simulink model "BuildingModelWithSolarLoadAndHVAC"  (R2025a)
settings: Solver=daessc  StartTime=0.0  StopTime=604800  FixedStep=60*15  MaxStep=60  RelTol=1e-3  AbsTol=1e-3
PreLoadFcn:
  | % WallModelParams
libraries: nesl_utility x12, fl_lib x6, slpidlib x1
(part 1 of 2)
CloseFcn:
  | % clear flow out roomHeight wall win
settings Model: Creator=vikrants  LastModifiedBy=vikrants
settings SolverCC: AutoScaleAbsTol=off  NumberNewtonIterations=3.0  AlgebraicLoopSolver=TrustRegion  MaxZcPerStep=1.0
settings DebuggingCC: UnconnectedInputMsg=warning  UnconnectedOutputMsg=warning  UnconnectedLineMsg=warning  SymbolicDimsDataTypeCodeGenerationDiagnostic=none
settings ModelReferenceCC: EnableRefExpFcnMdlSchedulingChecks=on
settings SFSimCC: CustomCodeUndefinedFunction=UseInterfaceOnly
settings RTWCC: GPUComputeCapability=3.5  DLArmComputeVersion=19.05
settings SimscapeCC: SimscapeLogType=all  SimscapeLogSimulationStatistics=on  SimscapeLogDataHistory=10000.0  SimscapeMultithreadedCompilation=off

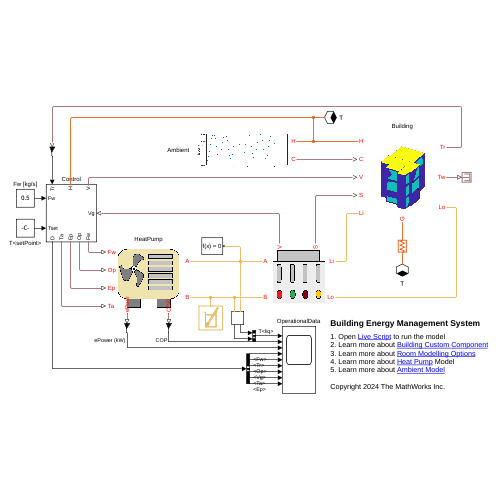
[thumbnail: Simulink's stored preview of the top-level diagram]
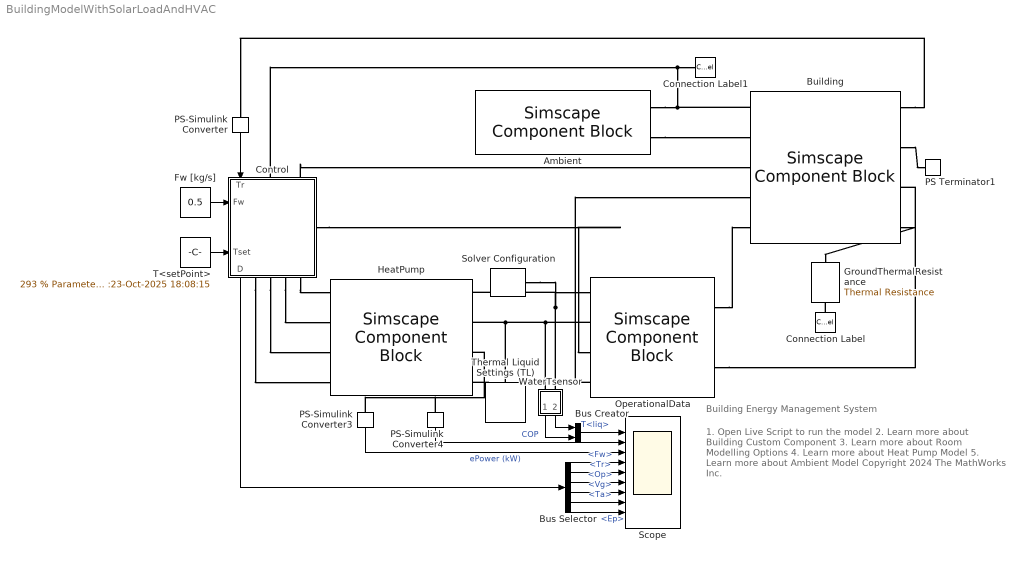
== system BuildingModelWithSolarLoadAndHVAC ==
  note: 1. Open Live Script to run the model
      | 2. Learn more about Building Custom Component
      | 3. Learn more about Room Modelling Options
      | 4. Learn more about Heat Pump Model
      | 5. Learn more about Ambient Model
      |
      | Copyright 2024 The MathWorks Inc.
  note: Building Energy Management System
  Ambient : SimscapeComponentBlock  SourceFile=EnvModel  ComponentPath=EnvModel  ComponentVariants="[\"EnvModel\"]"  ComponentVariantNames="[\"EnvModel\"]"  ClassName=EnvModel  SchemaVersion=1  listOfDays="[1  2  3  4  5  6  7] % Parameterized on :23-Oct-2025 18:08:15"  sunrise="[28933.8374      28933.0124      28929.4904      28923.2682      28914.3448      28902.7215       28888.402] % Parameterized on :23-Oct-2025 18:08:15 s"  sunset="[57466.1626      57466.9876      57470.5096      57476.7318      57485.6552      57497.2785       57511.598] % Parameterized on :23-Oct-2025 18:08:15 s"  startTime=3600 % Parameterized on :23-Oct-2025 18:08:15 s  avgDayTvec="[303  303  303  303  303  303  303] % Parameterized on :23-Oct-2025 18:08:15 K"  pcDayTvar=1 % Parameterized on :23-Oct-2025 18:08:15  avgNightTvec="[299  299  299  299  299  299  299] % Parameterized on :23-Oct-2025 18:08:15 K"  pcNightTvar=1 % Parameterized on :23-Oct-2025 18:08:15  cloudData=cloudCoverOptions.daily  cloudCoverVal="[0  0  0  0  0  0  0] % Parameterized on :23-Oct-2025 18:08:15"
      settings: CopyFcn=simscape.sscblock.internal.componentBlockCallback(gcbh,'COPY')  PreCopyFcn=simscape.sscblock.internal.componentBlockCallback(gcbh,'PRECOPY')  PreDeleteFcn=simscape.sscblock.internal.componentBlockCallback(gcbh,'PREDELETE')  InternalSimscapePortConfiguration="{\"Bottom\":[],\"Left\":[],\"Right\":[{\"id\":\"A\",\"label\":\"H\",\"type\":\"foundation.thermal.thermal\"},{\"id\":\"cloud\",\"label\":\"C\",\"type\":\"output\"}],\"Top\":[]}"
      mask Type: EnvModel
  Building : SimscapeComponentBlock  SourceFile=BuildingModel  ComponentPath=BuildingModel  ComponentVariants="[\"BuildingModel\"]"  ComponentVariantNames="[\"BuildingModel\"]"  ClassName=BuildingModel  SchemaVersion=1  nApts=3 % Parameterized on :23-Oct-2025 18:08:15  nRooms=5 % Parameterized on :23-Oct-2025 18:08:15  roomVolMat=[22.6534772736 39.6435852288 13.59208636416 9.9108963072 5.6633693184;22.6534772736 39.6435852288 13.59208636416 9.9108963072 5.6633693184;22.6534772736 39.6435852288 13.59208636416 9.9108963072 5.6633693184] % Parameterized on :23-Oct-2025 18:08:15 m^3  roomConnMat=[1 1 1 2 1.9235928 0.75;1 1 1 3 7.1789544 0.5;1 1 1 4 6.2816232 1;1 1 1 5 1.79493672 0.5;1 2 1 3 0.48121824 1;1 2 1 4 0.9614916 0.75;1 3 1 5 1.20210072 1;2 1 2 2 1.9235928 0.75;2 1 2 3 7.1789544 0.5;2 1 2 4 6.2816232 1;2 1 2 5 1.79493672 0.5;2 2 2 3 0.48121824 1;2 2 2 4 0.9614916 0.75;2 3 2 5 1.20210072 1;3 1 3 2 1.9235928 0.75;3 1 3 3 7.1789544 0.5;3 1 3 4 6.2816232 1;3 1 3 5 1.79493672 0.5;3 2 3 3 0.48121824 1;3 2 3 4 0.9614916 0.75;3 3 3 5 1.20210072 1] % Parameterized on :23-Oct-2025 18:08:15  floorConnMat=[1 1 2 1 7.43224 1;1 2 2 2 13.0064 1;1 3 2 3 4.45935 1;1 4 2 4 3.25161 1;1 5 2 5 1.85806 1;2 1 3 1 7.43224 1;2 2 3 2 13.0064 1;2 3 3 3 4.45935 1;2 4 3 4 3.25161 1;2 5 3 5 1.85806 1] % Parameterized on :23-Oct-2025 18:08:15  roomEnvConnMat=[1 1 1 2.22966 5.20254 0;1 1 2 1.393545 4.64515 0;1 1 4 1.85806 0 0;1 2 1 0 13.0064 0;1 2 2 9.2903 0 0;1 2 3 3.90192 9.10448 0;1 2 4 4.64515 4.64515 0;1 3 1 0.929051914 0 0;1 3 3 1.11484 3.90194 0;1 3 4 2.22966 5.20254 0;1 4 1 4.6452 0 0;1 4 2 4.55224 1.95096 0;1 4 3 0.92904 0 0;1 4 4 1.393570728 3.2516 0;1 5 1 4.6452 0 0;1 5 2 1.85805 0 0;1 5 3 0.92904 0 0;1 5 4 1.48644 2.22966 0;2 1 1 2.22966 5.20254 0;2 1 2 1.393545 4.64515 0;2 1 4 1.85806 0 0;2 2 1 0 13.0064 0;2 2 2 9.2903 0 0;2 2 3 3.90192 9.10448 0;2 2 4 4.64515 4.64515 0;2 3 1 0.929051914 0 0;2 3 3 1.11484 3.90194 0;2 3 4 2.22966 5.20254 0;2 4 1 4.6452 0 0;2 4 2 4.55224 1.95096 0;2 4 3 0.92904 0 0;2 4 4 1.393570728 3.2516 0;2 5 1 4.6452 0 0;2 5 2 1.85805 0 0;2 5 3 0.92904 0 0;2 5 4 1.48644 2.22966 0;3 1 1 2.22966 5.20254 0;3 1 2 1.393545 4.64515 0;3 1 4 1.85806 0 0;3 2 1 0 13.0064 0;3 2 2 9.2903 0 0;3 2 3 3.90192 9.10448 0;3 2 4 4.64515 4.64515 0;3 3 1 0.929051914 0 0;3 3 3 1.11484 3.90194 0;3 3 4 2.22966 5.20254 0;3 4 1 4.6452 0 0;3 4 2 4.55224 1.95096 0;3 4 3 0.92904 0 0;3 4 4 1.393570728 3.2516 0;3 5 1 4.6452 0 0;3 5 2 1.85805 0 0;3 5 3 0.92904 0 0;3 5 4 1.48644 2.22966 0] % Parameterized on :23-Oct-2025 18:08:15  roomEnvSolarRad=[0 0 0 0 0 0 0 0 0 0 0 93.65116 177.3749 198.6853 136.8637 0 0 0 0 0 0 0 0 0 0 0 0 0 0 0 0 0 0 0 0 94.86252 178.682 199.7233 137.414 0 0 0 0 0 0 0 0 0 0 0 0 0 0 0 0 0 0 0 0 96.10373 180.0564 200.8599 138.0853 0 0 0 0 0 0 0 0 0 0 0 0 0 0 0 0 0 0 0 0 97.37456 181.498 202.0955 138.8786 0 0 0 0 0 0 0 0 0 0 0 0 0 0 0 0 0 0 0 0 98.67471 183.0067 203.4304 139.7945 0 0 0 0 0 0 0 0 0 0 0 0 0 0 0 0 0 0 0 0 100.0039 184.5824 204.8647 140.834 0 0 0 0 0 0 0 0 0 0 0 0 0 0 0 0 0 0 0 0 101.3617 186.2247 206.3988 141.9976 0 0 0 0 0 0 0 0 0 0;0 0 0 0 0 0 0 0 0 0 0 0 0 0 0 0 0 0 0 0 0 0 0 0 0 0 0 0 0 0 0 0 0 0 0 0 0 0 0 0 0 0 0 0 0 0 0 0 0 0 0 0 0 0 0 0 0 0 0 0 0 0 0 0 0 0 0 0 0 0 0 0 0 0 0 0 0 0 0 0 0 0 0 0 0 0 0 0 0 0 0 0 0 0 0 0 0 0 0 0 0 0 0 0 0 0 0 0 0 0 0 0 0 0 0 0 0 0 0 0 0 0 0 0 0 0 0 0 0 0 0 0 0 0 0 0 0 0 0 0 0 0 0 0 0 0 0 0 0 0 0 0 0 0 0 0 0 0 0 0 0 0 0 0 0 0 0 0 0;0 0 0 0 0 0 0 0 142.8462 239.0062 293.6475 287.8589 224.8602 132.4751 48.80781 0 0 0 0 0 0 0 0 0 0 0 0 0 0 0 0 0 144.7366 240.8153 295.1148 288.755 225.1512 132.3647 48.62846 0 0 0 0 0 0 0 0 0 0 0 0 0 0 0 0 0 146.7023 242.7125 296.6788 289.7448 225.5201 132.3084 48.48171 0 0 0 0 0 0 0 0 0 0 0 0 0 0 0 0 0 148.7418 244.6967 298.3387 290.8281 225.9666 132.3058 48.36703 0 0 0 0 0 0 0 0 0 0 0 0 0 0 0 0 0 150.8536 246.7667 300.0937 292.0043 226.4904 132.3564 48.28381 0 0 0 0 0 0 0 0 0 0 0 0 0 0 0 0 0 153.0361 248.9213 301.9431 293.273 227.0912 132.4599 48.23142 0 0 0 0 0 0 0 0 0 0 0 0 0 0 0 0 0 155.2877 251.1593 303.886 294.6337 227.7686 132.6158 48.20913 0 0 0 0 0 0 0 0 0 0;0 0 0 0 0 0 0 0 0 0 0 93.65116 177.3749 198.6853 136.8637 0 0 0 0 0 0 0 0 0 0 0 0 0 0 0 0 0 0 0 0 94.86252 178.682 199.7233 137.414 0 0 0 0 0 0 0 0 0 0 0 0 0 0 0 0 0 0 0 0 96.10373 180.0564 200.8599 138.0853 0 0 0 0 0 0 0 0 0 0 0 0 0 0 0 0 0 0 0 0 97.37456 181.498 202.0955 138.8786 0 0 0 0 0 0 0 0 0 0 0 0 0 0 0 0 0 0 0 0 98.67471 183.0067 203.4304 139.7945 0 0 0 0 0 0 0 0 0 0 0 0 0 0 0 0 0 0 0 0 100.0039 184.5824 204.8647 140.834 0 0 0 0 0 0 0 0 0 0 0 0 0 0 0 0 0 0 0 0 101.3617 186.2247 206.3988 141.9976 0 0 0 0 0 0 0 0 0 0;0 0 0 0 0 0 0 0 0 0 0 0 0 0 0 0 0 0 0 0 0 0 0 0 0 0 0 0 0 0 0 0 0 0 0 0 0 0 0 0 0 0 0 0 0 0 0 0 0 0 0 0 0 0 0 0 0 0 0 0 0 0 0 0 0 0 0 0 0 0 0 0 0 0 0 0 0 0 0 0 0 0 0 0 0 0 0 0 0 0 0 0 0 0 0 0 0 0 0 0 0 0 0 0 0 0 0 0 0 0 0 0 0 0 0 0 0 0 0 0 0 0 0 0 0 0 0 0 0 0 0 0 0 0 0 0 0 0 0 0 0 0 0 0 0 0 0 0 0 0 0 0 0 0 0 0 0 0 0 0 0 0 0 0 0 0 0 0 0;0 0 0 0 0 0 0 0 0 0 0 0 0 0 0 0 0 0 0 0 0 0 0 0 0 0 0 0 0 0 0 0 0 0 0 0 0 0 0 0 0 0 0 0 0 0 0 0 0 0 0 0 0 0 0 0 0 0 0 0 0 0 0 0 0 0 0 0 0 0 0 0 0 0 0 0 0 0 0 0 0 0 0 0 0 0 0 0 0 0 0 0 0 0 0 0 0 0 0 0 0 0 0 0 0 0 0 0 0 0 0 0 0 0 0 0 0 0 0 0 0 0 0 0 0 0 0 0 0 0 0 0 0 0 0 0 0 0 0 0 0 0 0 0 0 0 0 0 0 0 0 0 0 0 0 0 0 0 0 0 0 0 0 0 0 0 0 0 0;0 0 0 0 0 0 0 0 142.8462 239.0062 293.6475 287.8589 224.8602 132.4751 48.80781 0 0 0 0 0 0 0 0 0 0 0 0 0 0 0 0 0 144.7366 240.8153 295.1148 288.755 225.1512 132.3647 48.62846 0 0 0 0 0 0 0 0 0 0 0 0 0 0 0 0 0 146.7023 242.7125 296.6788 289.7448 225.5201 132.3084 48.48171 0 0 0 0 0 0 0 0 0 0 0 0 0 0 0 0 0 148.7418 244.6967 298.3387 290.8281 225.9666 132.3058 48.36703 0 0 0 0 0 0 0 0 0 0 0 0 0 0 0 0 0 150.8536 246.7667 300.0937 292.0043 226.4904 132.3564 48.28381 0 0 0 0 0 0 0 0 0 0 0 0 0 0 0 0 0 153.0361 248.9213 301.9431 293.273 227.0912 132.4599 48.23142 0 0 0 0 0 0 0 0 0 0 0 0 0 0 0 0 0 155.2877 251.1593 303.886 294.6337 227.7686 132.6158 48.20913 0 0 0 0 0 0 0 0 0 0;0 0 0 0 0 0 0 0 0 0 0 93.65116 177.3749 198.6853 136.8637 0 0 0 0 0 0 0 0 0 0 0 0 0 0 0 0 0 0 0 0 94.86252 178.682 199.7233 137.414 0 0 0 0 0 0 0 0 0 0 0 0 0 0 0 0 0 0 0 0 96.10373 180.0564 200.8599 138.0853 0 0 0 0 0 0 0 0 0 0 0 0 0 0 0 0 0 0 0 0 97.37456 181.498 202.0955 138.8786 0 0 0 0 0 0 0 0 0 0 0 0 0 0 0 0 0 0 0 0 98.67471 183.0067 203.4304 139.7945 0 0 0 0 0 0 0 0 0 0 0 0 0 0 0 0 0 0 0 0 100.0039 184.5824 204.8647 140.834 0 0 0 0 0 0 0 0 0 0 0 0 0 0 0 0 0 0 0 0 101.3617 186.2247 206.3988 141.9976 0 0 0 0 0 0 0 0 0 0;0 0 0 0 0 0 0 0 0 0 0 0 0 0 0 0 0 0 0 ...(+22234 chars)] % Parameterized on :23-Oct-2025 18:08:15  floorGroundConn=[1 1 7.4322432;1 2 13.0064256;1 3 4.45934592;1 4 3.2516064;1 5 1.8580608] % Parameterized on :23-Oct-2025 18:08:15  roomModelOption=roomPhysicsOptions.roomRadiatorUF  roomRadiatorArea=[2.322576 3.2516064 1.8580608 1.6258032 1.161288;2.322576 3.2516064 1.8580608 1.6258032 1.161288;2.322576 3.2516064 1.8580608 1.6258032 1.161288] % Parameterized on :23-Oct-2025 18:08:15 m^2  roomUFPipingArea=[7.4322432 13.0064256 4.013411328 2.92644576 1.8580608;7.4322432 13.0064256 4.013411328 2.92644576 1.8580608;7.4322432 13.0064256 4.013411328 2.92644576 1.8580608] % Parameterized on :23-Oct-2025 18:08:15 m^2  roofEnvConnMat=[3 1 7.4322432;3 2 13.0064256;3 3 4.45934592;3 4 3.2516064;3 5 1.8580608] % Parameterized on :23-Oct-2025 18:08:15  roofEnvSolarRad=[0 0 0 0 0 0 0 0 135.3688 244.6002 318.0249 338.3299 301.6173 215.2339 101.2105 0 0 0 0 0 0 0 0 0 0 0 0 0 0 0 0 0 137.349 246.6202 319.7841 339.6663 302.4684 215.6179 101.2704 0 0 0 0 0 0 0 0 0 0 0 0 0 0 0 0 0 139.4098 248.7357 321.6488 341.1138 303.4312 216.1063 101.4179 0 0 0 0 0 0 0 0 0 0 0 0 0 0 0 0 0 141.55 250.9457 323.6182 342.672 304.5056 216.6994 101.653 0 0 0 0 0 0 0 0 0 0 0 0 0 0 0 0 0 143.7687 253.249 325.6913 344.3403 305.6916 217.3972 101.9758 0 0 0 0 0 0 0 0 0 0 0 0 0 0 0 0 0 146.0648 255.6446 327.8673 346.1181 306.9889 218.1999 102.3866 0 0 0 0 0 0 0 0 0 0 0 0 0 0 0 0 0 148.4371 258.1313 330.1451 348.0048 308.3973 219.1077 102.8853 0 0 0 0 0 0 0 0 0 0;0 0 0 0 0 0 0 0 135.3688 244.6002 318.0249 338.3299 301.6173 215.2339 101.2105 0 0 0 0 0 0 0 0 0 0 0 0 0 0 0 0 0 137.349 246.6202 319.7841 339.6663 302.4684 215.6179 101.2704 0 0 0 0 0 0 0 0 0 0 0 0 0 0 0 0 0 139.4098 248.7357 321.6488 341.1138 303.4312 216.1063 101.4179 0 0 0 0 0 0 0 0 0 0 0 0 0 0 0 0 0 141.55 250.9457 323.6182 342.672 304.5056 216.6994 101.653 0 0 0 0 0 0 0 0 0 0 0 0 0 0 0 0 0 143.7687 253.249 325.6913 344.3403 305.6916 217.3972 101.9758 0 0 0 0 0 0 0 0 0 0 0 0 0 0 0 0 0 146.0648 255.6446 327.8673 346.1181 306.9889 218.1999 102.3866 0 0 0 0 0 0 0 0 0 0 0 0 0 0 0 0 0 148.4371 258.1313 330.1451 348.0048 308.3973 219.1077 102.8853 0 0 0 0 0 0 0 0 0 0;0 0 0 0 0 0 0 0 135.3688 244.6002 318.0249 338.3299 301.6173 215.2339 101.2105 0 0 0 0 0 0 0 0 0 0 0 0 0 0 0 0 0 137.349 246.6202 319.7841 339.6663 302.4684 215.6179 101.2704 0 0 0 0 0 0 0 0 0 0 0 0 0 0 0 0 0 139.4098 248.7357 321.6488 341.1138 303.4312 216.1063 101.4179 0 0 0 0 0 0 0 0 0 0 0 0 0 0 0 0 0 141.55 250.9457 323.6182 342.672 304.5056 216.6994 101.653 0 0 0 0 0 0 0 0 0 0 0 0 0 0 0 0 0 143.7687 253.249 325.6913 344.3403 305.6916 217.3972 101.9758 0 0 0 0 0 0 0 0 0 0 0 0 0 0 0 0 0 146.0648 255.6446 327.8673 346.1181 306.9889 218.1999 102.3866 0 0 0 0 0 0 0 0 0 0 0 0 0 0 0 0 0 148.4371 258.1313 330.1451 348.0048 308.3973 219.1077 102.8853 0 0 0 0 0 0 0 0 0 0;0 0 0 0 0 0 0 0 135.3688 244.6002 318.0249 338.3299 301.6173 215.2339 101.2105 0 0 0 0 0 0 0 0 0 0 0 0 0 0 0 0 0 137.349 246.6202 319.7841 339.6663 302.4684 215.6179 101.2704 0 0 0 0 0 0 0 0 0 0 0 0 0 0 0 0 0 139.4098 248.7357 321.6488 341.1138 303.4312 216.1063 101.4179 0 0 0 0 0 0 0 0 0 0 0 0 0 0 0 0 0 141.55 250.9457 323.6182 342.672 304.5056 216.6994 101.653 0 0 0 0 0 0 0 0 0 0 0 0 0 0 0 0 0 143.7687 253.249 325.6913 344.3403 305.6916 217.3972 101.9758 0 0 0 0 0 0 0 0 0 0 0 0 0 0 0 0 0 146.0648 255.6446 327.8673 346.1181 306.9889 218.1999 102.3866 0 0 0 0 0 0 0 0 0 0 0 0 0 0 0 0 0 148.4371 258.1313 330.1451 348.0048 308.3973 219.1077 102.8853 0 0 0 0 0 0 0 0 0 0;0 0 0 0 0 0 0 0 135.3688 244.6002 318.0249 338.3299 301.6173 215.2339 101.2105 0 0 0 0 0 0 0 0 0 0 0 0 0 0 0 0 0 137.349 246.6202 319.7841 339.6663 302.4684 215.6179 101.2704 0 0 0 0 0 0 0 0 0 0 0 0 0 0 0 0 0 139.4098 248.7357 321.6488 341.1138 303.4312 216.1063 101.4179 0 0 0 0 0 0 0 0 0 0 0 0 0 0 0 0 0 141.55 250.9457 323.6182 342.672 304.5056 216.6994 101.653 0 0 0 0 0 0 0 0 0 0 0 0 0 0 0 0 0 143.7687 253.249 325.6913 344.3403 305.6916 217.3972 101.9758 0 0 0 0 0 0 0 0 0 0 0 0 0 0 0 0 0 146.0648 255.6446 327.8673 346.1181 306.9889 218.1999 102.3866 0 0 0 0 0 0 0 0 0 0 0 0 0 0 0 0 0 148.4371 258.1313 330.1451 348.0048 308.3973 219.1077 102.8853 0 0 0 0 0 0 0 0 0 0] % Parameterized on :23-Oct-2025 18:08:15  radiatorPipeGap=1e-2 m  radiatorPipeHydrDia=0.022 m  radiatorPipeArea=pi*(0.022^2)/4 m^2  UFPipeGap=1e-2 m  UFPipeHydrDia=0.015 m  UFPipeArea=pi*(0.015^2)/4 m^2  wallPropValue=wallPhysicsOptions.allWallNotSame  wallAbsorptivityValue=0.6  wallThicknessValue=.3 m  wallMaterialDenValue=2400 kg/m^3  wallMaterialCpValue=750 J/(K*kg)  wallThermalKValue=2 W/(K*m)  extWallAbsorptivityVal=0.6 % Parameterized on :23-Oct-2025 18:08:15  extWallThicknessVal=0.3 % Parameterized on :23-Oct-2025 18:08:15 m  extWallMaterialDenVal=2400 % Parameterized on :23-Oct-2025 18:08:15 kg/m^3  extWallMaterialCpVal=750 % Parameterized on :23-Oct-2025 18:08:15 J/(K*kg)  extWallThermalKVal=2 % Parameterized on :23-Oct-2025 18:08:15 W/(K*m)  intWallThicknessVal=0.3 % Parameterized on :23-Oct-2025 18:08:15 m  intWallMaterialDenVal=2400 % Parameterized on :23-Oct-2025 18:08:15 kg/m^3  intWallMaterialCpVal=750 % Parameterized on :23-Oct-2025 18:08:15 J/(K*kg)  intWallThermalKVal=2 % Parameterized on :23-Oct-2025 18:08:15 W/(K*m)  intFloorThicknessVal=0.3 % Parameterized on :23-Oct-2025 18:08:15 m  intFloorMaterialDenVal=2400 % Parameterized on :23-Oct-2025 18:08:15 kg/m^3  intFloorMaterialCpVal=750 % Parameterized on :23-Oct-2025 18:08:15 J/(K*kg)  intFloorThermalKVal=2 % Parameterized on :23-Oct-2025 18:08:15 W/(K*m)  roofAbsorptivityVal=0.6 % Parameterized on :23-Oct-2025 18:08:15  roofThicknessVal=0.3 % Parameterized on :23-Oct-2025 18:08:15 m  roofMaterialDenVal=2400 % Parameterized on :23-Oct-2025 18:08:15 kg/m^3  roofMaterialCpVal=750 % Parameterized on :23-Oct-2025 18:08:15 J/(K*kg)  roofThermalKVal=2 % Parameterized on :23-Oct-2025 18:08:15 W/(K*m)  winAbsorptivity=0.4 % Parameterized on :23-Oct-2025 18:08:15  winTransmissivity=0.2 % Parameterized on :23-Oct-2025 18:08:15  winThickness=0.01 % Parameterized on :23-Oct-2025 18:08:15 m  winMaterialDen=4000 % Parameterized on :23-Oct-2025 18:08:15 kg/m^3  winMaterialCp=840 % Parameterized on :23-Oct-2025 18:08:15 J/(K*kg)  winThermalK=1 % Parameterized on :23-Oct-2025 18:08:15 W/(K*m)  heatTransferPipeRoughness=1e-06 m  extToWallHTC=50 % Parameterized on :23-Oct-2025 18:08:15 W/(K*m^2)  intToRoomHTC=25 % Parameterized on :23-Oct-2025 18:08:15 W/(K*m^2)  iniTemperature=294.1 % Parameterized on :23-Oct-2025 18:08:15 K  airDensity=1.28 kg/m^3  airCp=700 J/(K*kg)  minArea=1e-10 m^2
      settings: CopyFcn=simscape.sscblock.internal.componentBlockCallback(gcbh,'COPY')  PreCopyFcn=simscape.sscblock.internal.componentBlockCallback(gcbh,'PRECOPY')  PreDeleteFcn=simscape.sscblock.internal.componentBlockCallback(gcbh,'PREDELETE')  InternalSimscapePortConfiguration="{\"Bottom\":[{\"id\":\"G\",\"label\":\"G\",\"type\":\"foundation.thermal.thermal\"}],\"Left\":[{\"id\":\"H\",\"label\":\"H\",\"type\":\"foundation.thermal.thermal\"},{\"id\":\"C\",\"label\":\"C\",\"type\":\"input\"},{\"id\":\"V\",\"label\":\"V\",\"type\":\"input\"},{\"id\":\"S\",\"label\":\"S\",\"type\":\"input\"},{\"id\":\"A\",\"label\":\"Li\",\"type\":\"foundation.thermal_liquid.thermal_liquid\"}],\"Right\":[{\"id\":\"roomTemp\",\"label\":\"Tr\",\"type\":\"output\"},{\"id\":\"wallTemp\",\"label\":\"Tw\",\"type\":\"output\"},{\"id\":\"B\",\"label\":\"Lo\",\"type\":\"foundation.thermal_liquid.thermal_liquid\"}],\"Top\":[]}"
      mask Type: BuildingModel
  Bus Creator : BusCreator  Inputs=2
  Bus Selector : BusSelector  OutputSignals=Fw,Tr,Op,Vg,Ta,Ep
  Connection Label : ConnectionLabel  Label=T
  Connection Label1 : ConnectionLabel  Label=T
  Control : Subsystem
      settings: PortSchema="{\"entries\":[{\"content\":{\"sides\":[{\"content\":{\"connectorIds\":[\"LConn1\"]},\"type\":\"ConnectorPlacement.EquallySpacedRectSide\",\"uuid\":\"3ed745ff-0b79-4fb7-8a1a-34583b4b790f\"},{\"content\":{\"connectorIds\":[\"In2\",\"In3\"],\"side\":\"RIGHT\"},\"type\":\"ConnectorPlacement.EquallySpacedRectSide\",\"uuid\":\"620bee4e-94f2-4040-b1cd-05a3221b3be9\"},{\"content\":{\"connectorIds\":[\"LConn2\",\"LConn3\",\"LConn4\",\"LConn5\",\"Out1\"],\"side\":\"TOP\"},\"type\":\"ConnectorPlacement.EquallySpacedRectSide\",\"uuid\":\"f68ff0b5-8e3a-4982-a173-63d19766a609\"},{\"content\":{\"connectorIds\":[\"RConn1\",\"RConn2\",\"In1\"],\"side\":\"BOTTOM\"},\"type\":\"ConnectorPlacement.EquallySpacedRectSide\",\"uuid\":\"2c8538cc-0234-4c65-909e-07f5b83fead8\"}]},\"type\":\"ConnectorPlacement.EquallySpacedConnector\",\"uuid\":\"126dfa7a-8255-403e-a375-633719ca790e\"}],\"packageUris\":[\"http://schema.mathworks.com/mf0/Connector/R2020b\"],\"version\":\"1.0\"}"
  Fw [kg/s] : Constant  Value=0.5
  GroundThermalResistance : fl_lib/Thermal/Thermal Elements/Thermal Resistance  resistance=100 % Parameterized on :23-Oct-2025 18:08:15 K/W  T_specify=off  T_priority=None  T=0 K  T_nominal_specify=off  T_nominal_value=1  T_nominal_unit=K  Q_specify=off  Q_priority=None  Q=0 W  Q_nominal_specify=off  Q_nominal_value=1  Q_nominal_unit=W
  HeatPump : SimscapeComponentBlock  SourceFile=HeatPumpModel  ComponentPath=HeatPumpModel  ComponentVariants="[\"HeatPumpModel\"]"  ComponentVariantNames="[\"HeatPumpModel\"]"  ClassName=HeatPumpModel  SchemaVersion=1  heatingCapacityA=10.17 kW  heatingCoPA=4.86  heatingCapacityB=10.12 kW  heatingCoPB=3.7  heatingCapacityC=10.17 kW  heatingCoPC=4.86  heatingCapacityD=10.12 kW  heatingCoPD=3.7  coolingCapacityE=10.55 kW  coolingCoPE=4.13  coolingCapacityF=6.9 kW  coolingCoPF=2.7  elecHeaterPower=2 kW  coilLen=1 m  coilDia=.05 m  coilArea=pi*(0.05^2)/4 m^2  initialT=299.8 K  initialP=.101325*2 MPa  expansionVol=0.01 m^3  nomDevOption=NominalConditionDeviationModel.enabled  modelOption=HeatPumpOptions.singleUnit  numHeatPumps=3  nominalFlow=0.5 kg/s  minWaterFlowRate=1e-3 kg/s  measTimelag=6 s  waterOpTempMin=281 K  waterOpTempMax=345 K  waterSpHeat=[4183, 4187, 4180, 4180, 4180, 4195] J/(K*kg)
      settings: CopyFcn=simscape.sscblock.internal.componentBlockCallback(gcbh,'COPY')  PreCopyFcn=simscape.sscblock.internal.componentBlockCallback(gcbh,'PRECOPY')  PreDeleteFcn=simscape.sscblock.internal.componentBlockCallback(gcbh,'PREDELETE')  InternalSimscapePortConfiguration="{\"Bottom\":[{\"id\":\"ePow\",\"label\":\"ePow\",\"type\":\"output\"},{\"id\":\"COP\",\"label\":\"COP\",\"type\":\"output\"}],\"Left\":[{\"id\":\"Fw\",\"label\":\"Fw\",\"type\":\"input\"},{\"id\":\"Op\",\"label\":\"Op\",\"type\":\"input\"},{\"id\":\"Ep\",\"label\":\"Ep\",\"type\":\"input\"},{\"id\":\"Ta\",\"label\":\"Ta\",\"type\":\"input\"}],\"Right\":[{\"id\":\"A\",\"label\":\"A\",\"type\":\"foundation.thermal_liquid.thermal_liquid\"},{\"id\":\"B\",\"label\":\"B\",\"type\":\"foundation.thermal_liquid.thermal_liquid\"}],\"Top\":[]}"
      mask Type: HeatPumpModel
  OperationalData : SimscapeComponentBlock  SourceFile=BuildingHVACOperation  ComponentPath=BuildingHVACOperation  ComponentVariants="[\"BuildingHVACOperation\"]"  ComponentVariantNames="[\"BuildingHVACOperation\"]"  ClassName=BuildingHVACOperation  SchemaVersion=1  roomModelOption=roomPhysicsOptions.roomRadiatorUF  opsParamBldg=[1 1 1 1 0 0 0;1 1 2 1 0 0 0;1 1 3 1 0 0 0;1 1 4 1 0 0 0;1 1 5 1 0 0 0;2 2 1 1 0 0 0;2 2 2 1 0 0 2;2 2 3 1 0 0 0;2 2 4 1 0 0 0;2 2 5 1 0 0 0;3 3 1 1 0 0 0;3 3 2 1 0 0 0;3 3 3 1 0 0 0;3 3 4 1 0 0 0;3 3 5 1 0 0 0;1 1 1 1 0 0 0;1 1 2 1 0 0 0;1 1 3 1 0 0 0;1 1 4 1 0 0 0;1 1 5 1 0 0 0;2 2 1 1 0 0 0;2 2 2 1 0 0 2;2 2 3 1 0 0 0;2 2 4 1 0 0 0;2 2 5 1 0 0 0;3 3 1 1 0 0 0;3 3 2 1 0 0 0;3 3 3 1 0 0 0;3 3 4 1 0 0 0;3 3 5 1 0 0 0;1 1 1 1 0 0 0;1 1 2 1 0 0 0;1 1 3 1 0 0 0;1 1 4 1 0 0 0;1 1 5 1 0 0 0;2 2 1 1 0 0 0;2 2 2 1 0 0 2;2 2 3 1 0 0 0;2 2 4 1 0 0 0;2 2 5 1 0 0 0;3 3 1 1 0 0 0;3 3 2 1 0 0 0;3 3 3 1 0 0 0;3 3 4 1 0 0 0;3 3 5 1 0 0 0;1 1 1 1 0 0 1;1 1 2 1 0 0 0;1 1 3 1 0 0 0;1 1 4 1 0 0 0;1 1 5 1 0 0 0;2 2 1 1 0 0 0;2 2 2 1 0 0 0;2 2 3 1 0 0 0;2 2 4 1 0 0 0;2 2 5 1 0 0 0;3 3 1 1 0 0 0;3 3 2 1 0 0 0;3 3 3 1 0 0 0;3 3 4 1 0 0 0;3 3 5 1 0 0 0;1 1 1 1 0 0 1;1 1 2 1 0 0 0;1 1 3 1 0 0 0;1 1 4 1 0 0 0;1 1 5 1 0 0 0;2 2 1 1 0 0 0;2 2 2 1 0 0 0;2 2 3 1 0 0 0;2 2 4 1 0 0 0;2 2 5 1 0 0 0;3 3 1 1 0 0 0;3 3 2 1 0 0 0;3 3 3 1 0 0 0;3 3 4 1 0 0 0;3 3 5 1 0 0 0;1 1 1 1 0 0 1;1 1 2 1 0 0 0;1 1 3 1 0 0 0;1 1 4 1 0 0 0;1 1 5 1 0 0 0;2 2 1 1 0 0 0;2 2 2 1 0 0 0;2 2 3 1 0 0 0;2 2 4 1 0 0 0;2 2 5 1 0 0 0;3 3 1 1 0 0 0;3 3 2 1 0 0 0;3 3 3 1 0 0 0;3 3 4 1 0 0 0;3 3 5 1 0 0 0;1 1 1 0 0 0 0;1 1 2 0 0 0 0;1 1 3 0 0 0 0;1 1 4 0 0 0 0;1 1 5 1 0 0 0;2 2 1 0 0 0 0;2 2 2 0 0 0 0;2 2 3 0 0 0 0;2 2 4 0 0 0 0;2 2 5 1 0 0 0;3 3 1 0 0 0 0;3 3 2 0 0 0 0;3 3 3 0 0 0 0;3 3 4 0 0 0 0;3 3 5 1 0 0 0;1 1 1 0 0 0 0;1 1 2 0 0 0 0;1 1 3 0 0 0 0;1 1 4 0 0 0 0;1 1 5 1 0 0 0;2 2 1 0 0 0 0;2 2 2 0 0 0 0;2 2 3 0 0 0 0;2 2 4 0 0 0 0;2 2 5 1 0 0 0;3 3 1 0 0 0 0;3 3 2 0 0 0 0;3 3 3 0 0 0 0;3 3 4 0 0 0 0;3 3 5 1 0 0 0;1 1 1 0 0 0 0;1 1 2 0 0 0 0;1 1 3 0 0 0 0;1 1 4 0 0 0 0;1 1 5 1 0 0 0;2 2 1 0 0 0 0;2 2 2 0 0 0 0;2 2 3 0 0 0 0;2 2 4 0 0 0 0;2 2 5 1 0 0 0;3 3 1 0 0 0 0;3 3 2 0 0 0 0;3 3 3 0 0 0 0;3 3 4 0 0 0 0;3 3 5 1 0 0 0;1 1 1 0 0 0 0;1 1 2 0 0 0 0;1 1 3 0 0 0 0;1 1 4 0 0 0 0;1 1 5 1 0 0 0;2 2 1 0 0 0 0;2 2 2 0 0 0 0;2 2 3 0 0 0 0;2 2 4 0 0 0 0;2 2 5 1 0 0 0;3 3 1 0 0 0 0;3 3 2 0 0 0 0;3 3 3 0 0 0 0;3 3 4 0 0 0 0;3 3 5 1 0 0 0;1 1 1 0 0 0 0;1 1 2 0 0 0 0;1 1 3 0 0 0 0;1 1 4 0 0 0 0;1 1 5 1 0 0 0;2 2 1 0 0 0 0;2 2 2 0 0 0 0;2 2 3 0 0 0 0;2 2 4 0 0 0 0;2 2 5 1 0 0 0;3 3 1 0 0 0 0;3 3 2 0 0 0 0;3 3 3 0 0 0 0;3 3 4 0 0 0 0;3 3 5 1 0 0 0;1 1 1 0 0 0 0;1 1 2 0 0 0 0;1 1 3 0 0 0 0;1 1 4 0 0 0 0;1 1 5 1 0 0 0;2 2 1 0 0 0 0;2 2 2 0 0 0 0;2 2 3 0 0 0 0;2 2 4 0 0 0 0;2 2 5 1 0 0 0;3 3 1 0 0 0 0;3 3 2 0 0 0 0;3 3 3 0 0 0 0;3 3 4 0 0 0 0;3 3 5 1 0 0 0;1 1 1 0 0 0 0;1 1 2 0 0 0 0;1 1 3 0 0 0 0;1 1 4 0 0 0 0;1 1 5 1 0 0 0;2 2 1 0 0 0 0;2 2 2 0 0 0 0;2 2 3 0 0 0 0;2 2 4 0 0 0 0;2 2 5 1 0 0 0;3 3 1 0 0 0 0;3 3 2 0 0 0 0;3 3 3 0 0 0 0;3 3 4 0 0 0 0;3 3 5 1 0 0 0;1 1 1 1 0 0 0;1 1 2 1 0 0 0;1 1 3 1 0 0 0;1 1 4 1 0 0 0;1 1 5 1 0 0 0;2 2 1 1 0 0 0;2 2 2 1 0 0 0;2 2 3 1 0 0 0;2 2 4 1 0 0 0;2 2 5 1 0 0 0;3 3 1 1 0 0 0;3 3 2 1 0 0 0;3 3 3 1 0 0 2;3 3 4 1 0 0 0;3 3 5 1 0 0 0;1 1 1 1 0 0 0;1 1 2 1 0 0 0;1 1 3 1 0 0 0;1 1 4 1 0 0 0;1 1 5 1 0 0 0;2 2 1 1 0 0 0;2 2 2 1 0 0 2;2 2 3 1 0 0 0;2 2 4 1 0 0 0;2 2 5 1 0 0 0;3 3 1 1 0 0 0;3 3 2 1 0 0 0;3 3 3 1 0 0 0;3 3 4 1 0 0 0;3 3 5 1 0 0 0;1 1 1 1 0 0 0;1 1 2 1 0 0 0;1 1 3 1 0 0 0;1 1 4 1 0 0 0;1 1 5 1 0 0 0;2 2 1 1 0 0 0;2 2 2 1 0 0 2;2 2 3 1 0 0 0;2 2 4 1 0 0 0;2 2 5 1 0 0 0;3 3 1 1 0 0 0;3 3 2 1 0 0 0;3 3 3 1 0 0 0;3 3 4 1 0 0 0;3 3 5 1 0 0 0;1 1 1 1 0 0 0;1 1 2 1 0 0 0;1 1 3 1 0 0 0;1 1 4 1 0 0 0;1 1 5 1 0 0 0;2 2 1 1 0 0 0;2 2 2 1 0 0 2;2 2 3 1 0 0 0;2 2 4 1 0 0 0;2 2 5 1 0 0 0;3 3 1 1 0 0 0;3 3 2 1 0 0 0;3 3 3 1 0 0 0;3 3 4 1 0 0 0;3 3 5 1 0 0 0;1 1 1 1 0 0 0;1 1 2 1 0 0 0;1 1 3 1 0 0 0;1 1 4 1 0 0 0;1 1 5 1 0 0 0;2 2 1 1 0 0 0;2 2 2 1 0 0 2;2 2 3 1 0 0 0;2 2 4 1 0 0 0;2 2 5 1 0 0 0;3 3 1 1 0 0 0;3 3 2 1 0 0 0;3 3 3 1 0 0 0;3 3 4 1 0 0 0;3 3 5 1 0 0 0;1 1 1 1 0 0 0;1 1 2 1 0 0 0;1 1 3 1 0 0 0;1 1 4 1 0 0 0;1 1 5 1 0 0 0;2 2 1 1 0 0 0;2 2 2 1 0 0 2;2 2 3 1 0 0 0;2 2 4 1 0 0 0;2 2 5 1 0 0 0;3 3 1 1 0 0 0;3 3 2 1 0 0 0;3 3 3 1 0 0 0;3 3 4 1 0 0 0;3 3 5 1 0 0 0;1 1 1 1 ...(+31492 chars)] % Parameterized on :23-Oct-2025 18:08:15  heatPerOccupant=50 W
      settings: CopyFcn=simscape.sscblock.internal.componentBlockCallback(gcbh,'COPY')  PreCopyFcn=simscape.sscblock.internal.componentBlockCallback(gcbh,'PRECOPY')  PreDeleteFcn=simscape.sscblock.internal.componentBlockCallback(gcbh,'PREDELETE')  InternalSimscapePortConfiguration="{\"Bottom\":[],\"Left\":[{\"id\":\"HPA\",\"label\":\"A\",\"type\":\"foundation.thermal_liquid.thermal_liquid\"},{\"id\":\"HPB\",\"label\":\"B\",\"type\":\"foundation.thermal_liquid.thermal_liquid\"}],\"Right\":[{\"id\":\"BldgA\",\"label\":\"Li\",\"type\":\"foundation.thermal_liquid.thermal_liquid\"},{\"id\":\"BldgB\",\"label\":\"Lo\",\"type\":\"foundation.thermal_liquid.thermal_liquid\"}],\"Top\":[{\"id\":\"Vg\",\"label\":\"V\",\"type\":\"output\"},{\"id\":\"Qr\",\"label\":\"S\",\"type\":\"output\"}]}"
      mask Type: BuildingHVACOperation
  PS Terminator1 : fl_lib/Physical Signals/Sinks/PS Terminator
  PS-Simulink Converter : nesl_utility/PS-Simulink Converter  PhysicalDomain=network_engine_domain  SubClassName=ps_output  LeftPortType=input  RightPortType=output  PseudoPeriodic=off  Frequencies=[]  VectorFormat=inherit  Unit=inherit  AffineConversion=off
  PS-Simulink Converter3 : nesl_utility/PS-Simulink Converter  PhysicalDomain=network_engine_domain  SubClassName=ps_output  LeftPortType=input  RightPortType=output  PseudoPeriodic=off  Frequencies=[]  VectorFormat=inherit  Unit=inherit  AffineConversion=off
  PS-Simulink Converter4 : nesl_utility/PS-Simulink Converter  PhysicalDomain=network_engine_domain  SubClassName=ps_output  LeftPortType=input  RightPortType=output  PseudoPeriodic=off  Frequencies=[]  VectorFormat=inherit  Unit=inherit  AffineConversion=off
  Scope : Scope  NumInputPorts=9
      settings: ActiveDisplayYMinimum=272.84809  ActiveDisplayYMaximum=305.90309  DataLoggingVariableName=BuildingModelScopeData
  Solver Configuration : nesl_utility/Solver Configuration  PhysicalDomain=network_engine_domain  SubClassName=solver  LeftPortType=input  RightPortType=generic  Tones=[]  Harmonics=[]  SimulateNoise=off  Profile=off  UseLocalSampling=off  EnableSwitchedLinearOptims=on  FrequencyDomain=off  UseCCode=off  RelTol=0.001  AbsTol=1e-06  MinStep=1e-09  ToWorkspace=off  RevertToSquareIcSolve=off  NumHomotopyIterations=100  PhasorMode=off  PhasorModeNumHarmonics=1  ConsistencySolver=NEWTON_XTOL_AFTER_FTOL  IndexReductionMethod=DerivativeReplacement  DoDC=off  ResidualTolerance=1e-09  ConsistencyTolSource=GLOBAL  ConsistencyAbsTol=0.001  ConsistencyRelTol=0.001  ConsistencyTolFactor=0.001  UseLocalSolver=off  LocalSolverChoice=NE_BACKWARD_EULER_ADVANCER  ResolveIndetEquations=on  FunctionEvalNumThread=1  LocalSolverSampleTime=3600  DoFixedCost=off  MaxNonlinIter=3  MaxModeIter=2  ComputeImpulses=off  ImpulseIterations=2  LinearAlgebra=auto  LinearAlgebraNumThread=0  EquationFormulation=NE_TIME_EF  DelaysMemoryBudget=1024  AutomaticFiltering=on  FilteringTimeConstant=0.001  PartitionStorageMethod=AS_NEEDED  PartitionMemoryBudget=1024  PartitionMethod=ROBUST  MultibodyUseLocalSolver=off  MultibodyLocalSolverChoice=ODE1  MultibodyLocalSolverSampleTime=0.001
  T<setPoint> : Constant  Value=293 % Parameterized on :23-Oct-2025 18:08:15
  Thermal Liquid Settings (TL) : fl_lib/Thermal Liquid/Utilities/Thermal Liquid Settings (TL)  table_dimensions=foundation.enum.table_dimensions_TL.two_dimensional  T_TLU=[273.1600 : 10 : 373.16]' K  p_TLU=[0.01, 0.1, 5 : 5 : 50] MPa  p_atm=0.101325 MPa  pT_region_flag=foundation.enum.pT_region_TL.min_max  T_min=273.16 K  T_max=363.16 K  p_min=0.05 MPa  p_max=50 MPa  T_min_1D=273.16 K  T_max_1D=363.16 K  p_min_1D=0.05 MPa  p_max_1D=50 MPa  pT_validity_TLU=[1, 1, 1, 1, 1, 1, 1, 1, 1, 1, 1, 1; 1, 1, 1, 1, 1, 1, 1, 1, 1, 1, 1, 1; 1, 1, 1, 1, 1, 1, 1, 1, 1, 1, 1, 1; 1, 1, 1, 1, 1, 1, 1, 1, 1, 1, 1, 1; 1, 1, 1, 1, 1, 1, 1, 1, 1, 1, 1, 1; 0, 1, 1, 1, 1, 1, 1, 1, 1, 1, 1, 1; 0, 1, 1, 1, 1, 1, 1, 1, 1, 1, 1, 1; 0, 1, 1, 1, 1, 1, 1, 1, 1, 1, 1, 1; 0, 1, 1, 1, 1, 1, 1, 1, 1, 1, 1, 1; 0, 1, 1, 1, 1, 1, 1, 1, 1, 1, 1, 1; 0, 0, 1, 1, 1, 1, 1, 1, 1, 1, 1, 1]  properties_range_check=simscape.enum.assert.action.error  rho_parameterization_2D=foundation.enum.rho_parameterization_2D.rho_beta_alpha  rho_parameterization_1D=foundation.enum.rho_parameterization_1D.rho_vector  rho_TLU=[999.7973, 999.8431, 1002.3216, 1004.8218, 1007.293, 1009.7358, 1012.1506, 1014.5379, 1016.8979, 1019.2311, 1021.538, 1023.8188; 999.6579, 999.7009, 1002.0303, 1004.382, 1006.7084, 1009.0101, 1011.2874, 1013.5407, 1015.7703, 1017.9766, 1020.1599, 1022.3206; 998.1632, 998.2045, 1000.4375, 1002.6924, 1004.9239, 1007.1324, 1009.3183, 1011.4819, 1013.6236, 1015.7438, 1017.8428, 1019.921; 995.6057, 995.6458, 997.8186, 1000.0128, 1002.1841, 1004.3332, 1006.4603, 1008.566, 1010.6505, 1012.7144, 1014.758, 1016.7815; 992.1724, 992.2119, 994.3513, 996.5113, 998.6484, 1000.7633, 1002.8563, 1004.928, 1006.9788, 1009.009, 1011.0192, 1013.0097; 988.02, 988.0299, 990.1568, 992.3035, 994.4268, 996.5273, 998.6056, 1000.6622, 1002.6976, 1004.7123, 1006.7067, 1008.6813; 983.18, 983.1901, 985.3217, 987.4721, 989.5983, 991.7008, 993.7803, 995.8374, 997.8726, 999.8864, 1001.8795, 1003.8522; 977.75, 977.7583, 979.9094, 982.0783, 984.2216, 986.34, 988.4343, 990.505, 992.5529, 994.5786, 996.5825, 998.5654; 971.77, 971.7836, 973.9673, 976.1678, 978.3409, 980.4876, 982.6087, 984.7049, 986.7768, 988.8254, 990.8511, 992.8545; 965.26, 965.3023, 967.5311, 969.7753, 971.9901, 974.1764, 976.3354, 978.4676, 980.5741, 982.6556, 984.7129, 986.7465; 958.62, 958.6315, 960.627, 962.9267, 965.1944, 967.4314, 969.6387, 971.8173, 973.9681, 976.0921, 978.19, 980.2628] kg/m^3  beta_TLU=[1.9649, 1.9654, 1.9929, 2.0213, 2.0499, 2.0787, 2.1078, 2.1372, 2.1668, 2.1966, 2.2268, 2.2572; 2.0913, 2.0918, 2.1191, 2.1471, 2.1752, 2.2036, 2.2322, 2.261, 2.2899, 2.3191, 2.3485, 2.3781; 2.1786, 2.1791, 2.2067, 2.235, 2.2634, 2.2919, 2.3206, 2.3494, 2.3784, 2.4075, 2.4367, 2.4661; 2.2332, 2.2337, 2.2619, 2.2908, 2.3197, 2.3487, 2.3778, 2.407, 2.4363, 2.4657, 2.4951, 2.5246; 2.26, 2.2605, 2.2895, 2.3191, 2.3487, 2.3784, 2.4081, 2.4378, 2.4675, 2.4973, 2.5272, 2.5571; 2.2638, 2.2638, 2.2936, 2.324, 2.3544, 2.3848, 2.4151, 2.4455, 2.4758, 2.5062, 2.5365, 2.5669; 2.2472, 2.2472, 2.2779, 2.3092, 2.3403, 2.3715, 2.4025, 2.4336, 2.4646, 2.4955, 2.5264, 2.5573; 2.214, 2.214, 2.2455, 2.2776, 2.3096, 2.3415, 2.3733, 2.405, 2.4367, 2.4683, 2.4998, 2.5313; 2.1668, 2.1668, 2.1992, 2.2321, 2.2649, 2.2976, 2.3301, 2.3626, 2.3949, 2.4272, 2.4593, 2.4914; 2.1081, 2.1081, 2.1413, 2.175, 2.2086, 2.2421, 2.2754, 2.3085, 2.3415, 2.3744, 2.4072, 2.4399; 2.0494, 2.0494, 2.0739, 2.1084, 2.1428, 2.177, 2.211, 2.2449, 2.2786, 2.3121, 2.3455, 2.3788] GPa  alpha_TLU=1e-4 * [-.679, -.676, -.49, -.307, -.13, .041, .206, .365, .519, .668, .811, .949; .878, .881, .998, 1.114, 1.227, 1.337, 1.445, 1.549, 1.651, 1.75, 1.846, 1.939; 2.068, 2.069, 2.141, 2.213, 2.283, 2.352, 2.42, 2.486, 2.551, 2.614, 2.676, 2.736; 3.034, 3.035, 3.074, 3.113, 3.152, 3.191, 3.229, 3.267, 3.305, 3.341, 3.377, 3.413; 3.855, 3.856, 3.87, 3.884, 3.899, 3.914, 3.93, 3.946, 3.961, 3.977, 3.993, 4.009; 4.578, 4.578, 4.572, 4.566, 4.562, 4.558, 4.555, 4.552, 4.55, 4.549, 4.548, 4.547; 5.233, 5.233, 5.209, 5.186, 5.165, 5.144, 5.125, 5.107, 5.09, 5.074, 5.059, 5.045; 5.84, 5.84, 5.801, 5.762, 5.725, 5.691, 5.657, 5.625, 5.595, 5.566, 5.538, 5.512; 6.414, 6.414, 6.36, 6.307, 6.256, 6.208, 6.161, 6.117, 6.074, 6.033, 5.994, 5.956; 6.967, 6.967, 6.898, 6.831, 6.766, 6.705, 6.646, 6.589, 6.535, 6.482, 6.432, 6.384; 7.519, 7.519, 7.423, 7.342, 7.264, 7.189, 7.118, 7.049, 6.983, 6.92, 6.859, 6.8] 1/K  rho_TLU_2=[999.7973, 999.8431, 1002.3216, 1004.8218, 1007.293, 1009.7358, 1012.1506, 1014.5379, 1016.8979, 1019.2311, 1021.538, 1023.8188; 999.6579, 999.7009, 1002.0303, 1004.382, 1006.7084, 1009.0101, 1011.2874, 1013.5407, 1015.7703, 1017.9766, 1020.1599, 1022.3206; 998.1632, 998.2045, 1000.4375, 1002.6924, 1004.9239, 1007.1324, 1009.3183, 1011.4819, 1013.6236, 1015.7438, 1017.8428, 1019.921; 995.6057, 995.6458, 997.81864, 1000.0128, 1002.1841, 1004.3332, 1006.4603, 1008.566, 1010.6505, 1012.7144, 1014.758, 1016.7815; 992.1724, 992.2119, 994.3513, 996.5113, 998.6484, 1000.7633, 1002.8563, 1004.928, 1006.9788, 1009.009, 1011.0192, 1013.0097; 988.02, 988.0299, 990.1568, 992.3035, 994.4268, 996.5273, 998.6056, 1000.6622, 1002.6976, 1004.7123, 1006.7067, 1008.6813; 983.18, 983.1901, 985.3217, 987.4721, 989.5983, 991.7008, 993.7803, 995.8374, 997.8726, 999.8864, 1001.8795, 1003.8522; 977.75, 977.7583, 979.9094, 982.0783, 984.2216, 986.34, 988.4343, 990.505, 992.5529, 994.5786, 996.5825, 998.5654; 971.77, 971.7836, 973.9673, 976.1678, 978.3409, 980.4876, 982.6087, 984.7049, 986.7768, 988.8254, 990.8511, 992.8545; 965.26, 965.3023, 967.5311, 969.7753, 971.9901, 974.1764, 976.3354, 978.4676, 980.5741, 982.6556, 984.7129, 986.7465; 958.62, 958.6315, 960.627, 962.9267, 965.1944, 967.4314, 969.6387, 971.8173, 973.9681, 976.0921, 978.19, 980.2628] kg/m^3  rho_ref_3=998.21 kg/m^3  T_ref_3=293.16 K  p_ref_3=0.101325 MPa  beta_const_3=2.1791 GPa  alpha_const_3=2.0691e-4 1/K  rho_TLU_4=[999.84; 999.7; 998.2; 995.65; 992.21; 988.03; 983.19; 977.76; 971.78; 965.3; 958.8] kg/m^3  beta_const_4=2.1791 GPa  p_ref_4=0.101325 MPa  rho_ref_5=998.21 kg/m^3  T_ref_5=293.16 K  p_ref_5=0.101325 MPa  beta_const_5=2.1791 GPa  alpha_const_5=2.0691e-4 1/K  u_parameterization_2D=foundation.enum.u_parameterization_2D.u_cp  u_parameterization_1D=foundation.enum.u_parameterization_1D.u  u_TLU=[.0002, .0018, .086, .1588, .219, .267, .3034, .3288, .3436, .3483, .3435, .3294; 42.062, 42.06, 41.935, 41.804, 41.668, 41.527, 41.382, 41.233, 41.081, 40.924, 40.763, 40.599; 83.953, 83.948, 83.651, 83.349, 83.049, 82.749, 82.451, 82.153, 81.856, 81.56, 81.265, 80.971; 125.77, 125.76, 125.31, 124.86, 124.41, 123.97, 123.53, 123.1, 122.68, 122.25, 121.84, 121.42; 167.57, 167.56, 166.96, 166.37, 165.79, 165.21, 164.65, 164.09, 163.54, 163, 162.46, 161.94; 209.36, 209.36, 208.63, 207.9, 207.19, 206.48, 205.79, 205.11, 204.45, 203.79, 203.14, 202.5; 251.19, 251.19, 250.33, 249.47, 248.62, 247.79, 246.98, 246.18, 245.39, 244.62, 243.86, 243.12; 293.06, 293.06, 292.07, 291.07, 290.1, 289.14, 288.2, 287.28, 286.38, 285.49, 284.62, 283.77; 334.99, 334.99, 333.86, 332.73, 331.63, 330.54, 329.48, 328.44, 327.41, 326.41, 325.43, 324.46; 377, 377, 375.73, 374.46, 373.22, 372, 370.81, 369.64, 368.5, 367.38, 366.27, 365.19; 419.01, 419.01, 417.69, 416.27, 414.89, 413.54, 412.21, 410.91, 409.64, 408.4, 407.17, 405.98] kJ/kg  cp_TLU=[4.2199, 4.2194, 4.1957, 4.1726, 4.1508, 4.13, 4.1103, 4.0916, 4.0738, 4.0569, 4.0408, 4.0254; 4.1955, 4.1951, 4.1769, 4.1592, 4.1422, 4.1259, 4.1103, 4.0954, 4.0812, 4.0676, 4.0545, 4.0421; 4.1843, 4.184, 4.169, 4.1543, 4.1401, 4.1264, 4.1133, 4.1007, 4.0885, 4.0768, 4.0656, 4.0548; 4.1801, 4.1798, 4.1667, 4.1538, 4.1413, 4.1293, 4.1177, 4.1064, 4.0956, 4.0851, 4.075, 4.0653; 4.1796, 4.1794, 4.1675, 4.1558, 4.1444, 4.1334, 4.1227, 4.1123, 4.1023, 4.0926, 4.0832, 4.0741; 4.1813, 4.1813, 4.1702, 4.1592, 4.1484, 4.138, 4.1279, 4.1181, 4.1086, 4.0993, 4.0903, 4.0816; 4.185, 4.185, 4.1742, 4.1636, 4.1532, 4.1432, 4.1334, 4.1239, 4.1146, 4.1056, 4.0969, 4.0884; 4.1901, 4.1901, 4.1795, 4.169, 4.1588, 4.1489, 4.1393, 4.1299, 4.1207, 4.1118, 4.1032, 4.0947; 4.1968, 4.1968, 4.1862, 4.1757, 4.1655, 4.1555, 4.1458, 4.1364, 4.1273, 4.1183, 4.1096, 4.1012; 4.2052, 4.2052, 4.1944, 4.1837, 4.1733, 4.1632, 4.1534, 4.1438, 4.1345, 4.1255, 4.1166, 4.108; 4.2136, 4.2136, 4.2045, 4.1935, 4.1828, 4.1724, 4.1623, 4.1524, 4.1429, 4.1335, 4.1245, 4.1157] kJ/(K*kg)  u_TLU_2=[.0002, .0018, .086, .1588, .219, .267, .3034, .3288, .3436, .3483, .3435, .3294; 42.062, 42.06, 41.935, 41.804, 41.668, 41.527, 41.382, 41.233, 41.081, 40.924, 40.763, 40.599; 83.953, 83.948, 83.651, 83.349, 83.049, 82.749, 82.451, 82.153, 81.856, 81.56, 81.265, 80.971; 125.77, 125.76, 125.31, 124.86, 124.41, 123.97, 123.53, 123.1, 122.68, 122.25, 121.84, 121.42; 167.57, 167.56, 166.96, 166.37, 165.79, 165.21, 164.65, 164.09, 163.54, 163, 162.46, 161.94; 209.36, 209.36, 208.63, 207.9, 207.19, 206.48, 205.79, 205.11, 204.45, 203.79, 203.14, 202.5; 251.19, 251.19, 250.33, 249.47, 248.62, 247.79, 246.98, 246.18, 245.39, 244.62, 243.86, 243.12; 293.06, 293.06, 292.07, 291.07, 290.1, 289.14, 288.2, 287.28, 286.38, 285.49, 284.62, 283.77; 334.99, 334.99, 333.86, 332.73, 331.63, 330.54, 329.48, 328.44, 327.41, 326.41, 325.43, 324.46; 377, 377, 375.73, 374.46, 373.22, 372, 370.81, 369.64, 368.5, 367.38, 366.27, 365.19; 419.01, 419.01, 417.69, 416.27, 414.89, 413.54, 412.21, 410.91, 409.64, 408.4, 407.17, 405.98] kJ/kg  cp_TLU_3=[4.2199, 4.2194, 4.1957, 4.1726, 4.1508, 4.13, 4.1103, 4.0916, 4.0738, 4.0569, 4.0408, 4.0254; 4.1955, 4.1951, 4.1769, 4.1592, 4.1422, 4.1259, 4.1103, 4.0954, 4.0812, 4.0676, 4.0545, 4.0421; 4.1843, 4.184, 4.169, 4.1543, 4.1401, 4.1264, 4.1133, 4.1007, 4.0885, 4.0768, 4.0656, 4.0548; 4.1801, 4.1798, 4.1667, 4.1538, 4.1413, 4.1293, 4.1177, 4.1064, 4.0956, 4.0851, 4.075, 4.0653; 4.1796, 4.1794, 4.1675, 4.1558, 4.1444, 4.1334, 4.1227, 4.1123, 4.1023, 4.0926, 4.0832, 4.0741; 4.1813, 4.1813, 4.1702, 4.1592, 4.1484, 4.138, 4.1279, 4.1181, 4.1086, 4.0993, 4.0903, 4.0816; 4.185, 4.185, 4.1742, 4.1636, 4.1532, 4.1432, 4.1334, 4.1239, 4.1146, 4.1056, 4.0969, 4.0884; 4.1901, 4.1901, 4.1795, 4.169, 4.1588, 4.1489, 4.1393, 4.1299, 4.1207, 4.1118, 4.1032, 4.0947; 4.1968, 4.1968, 4.1862, 4.1757, 4.1655, 4.1555, 4.1458, 4.1364, 4.1273, 4.1183, 4.1096, 4.1012; 4.2052, 4.2052, 4.1944, 4.1837, 4.1733, 4.1632, 4.1534, 4.1438, 4.1345, 4.1255, 4.1166, 4.108; 4.2136, 4.2136, 4.2045, 4.1935, 4.1828, 4.1724, 4.1623, 4.1524, 4.1429, 4.1335, 4.1245, 4.1157] kJ/(K*kg)  u_TLU_4=[.0018; 42.06; 83.948; 125.76; 167.56; 209.36; 251.19; 293.06; 334.99; 377; 418.01] kJ/kg  cp_TLU_5=[4.2199; 4.1955; 4.1843; 4.1801; 4.1796; 4.1813; 4.185; 4.1901; 4.1968; 4.2052; 4.2136] kJ/(K*kg)  nu_TLU=[1.7917, 1.7914, 1.7763, 1.7615, 1.7473, 1.7338, 1.7208, 1.7085, 1.6967, 1.6854, 1.6747, 1.6645; 1.3061, 1.3059, 1.2986, 1.2914, 1.2845, 1.2779, 1.2716, 1.2656, 1.2598, 1.2543, 1.2491, 1.2441; 1.0032, 1.0032, .9995, .9959, .9924, .9891, .9859, .9829, .9801, .9774, .9748, .9724; .8006, .8005, .7987, .797, .7953, .7937, .7922, .7908, .7894, .7881, .787, .7859; .6577, .6577, .657, .6562, .6555, .6548, .6543, .6537, .6532, .6528, .6523, .652; .553, .553, .5529, .5527, .5526, .5525, .5524, .5524, .5524, .5524, .5524, .5525; .4739, .4739, .4741, .4743, .4745, .4747, .475, .4753, .4755, .4758, .4762, .4765; .4127, .4127, .4131, .4135, .4139, .4143, .4148, .4152, .4157, .4162, .4167, .4172; .3643, .3643, .3648, .3654, .3659, .3665, .367, .3676, .3682, .3688, .3694, .37; .3254, .3254, .3261, .3267, .3273, .328, .3286, .3293, .3299, .3306, .3312, .3319; .2866, .2866, .2945, .2952, .2959, .2965, .2972, .2979, .2986, .2993, .3, .3007] mm^2/s  nu_TLU_2=[1.7917; 1.3061; 1.0032; .8006; .6577; .553; .4739; .4127; .3643; .3254; .2866] mm^2/s  k_TLU=[561.04, 561.09, 563.8, 566.56, 569.32, 572.08, 574.82, 577.54, 580.24, 582.92, 585.57, 588.18; 580.02, 580.07, 582.45, 584.88, 587.32, 589.75, 592.18, 594.61, 597.02, 599.42, 601.8, 604.16; 598.44, 598.48, 600.73, 603.03, 605.33, 607.64, 609.94, 612.24, 614.54, 616.82, 619.1, 621.36; 615.48, 615.52, 617.73, 620, 622.26, 624.54, 626.81, 629.07, 631.34, 633.6, 635.85, 638.09; 630.6, 630.64, 632.87, 635.15, 637.44, 639.72, 642.01, 644.29, 646.57, 648.84, 651.11, 653.36; 643.61, 643.61, 645.88, 648.21, 650.53, 652.86, 655.18, 657.51, 659.82, 662.14, 664.44, 666.74; 654.39, 654.39, 656.73, 659.12, 661.5, 663.89, 666.27, 668.65, 671.02, 673.38, 675.74, 678.09; 663.13, 663.13, 665.54, 668, 670.46, 672.91, 675.36, 677.8, 680.24, 682.67, 685.09, 687.5; 670.02, 670.02, 672.51, 675.05, 677.59, 680.12, 682.64, 685.16, 687.67, 690.17, 692.66, 695.14; 675.27, 675.27, 677.85, 680.48, 683.11, 685.73, 688.34, 690.94, 693.53, 696.11, 698.68, 701.24; 680.52, 680.52, 681.77, 684.5, 687.22, 689.94, 692.64, 695.34, 698.02, 700.69, 703.35, 706] mW/(K*m)  k_TLU_2=[561.04; 580.02; 598.44; 615.48; 630.6; 643.61; 654.39; 663.13; 670.02; 675.27; 680.52] mW/(K*m)
  WaterTsensor : Subsystem
      settings: PortSchema="{\"entries\":[{\"content\":{\"sides\":[{\"content\":{},\"type\":\"ConnectorPlacement.EquallySpacedRectSide\",\"uuid\":\"319169eb-d120-4e07-a592-0511c40eb7cc\"},{\"content\":{\"side\":\"RIGHT\"},\"type\":\"ConnectorPlacement.EquallySpacedRectSide\",\"uuid\":\"75da7174-b234-4c2f-a38c-b7daad4bd044\"},{\"content\":{\"connectorIds\":[\"LConn1\",\"LConn2\"],\"side\":\"TOP\"},\"type\":\"ConnectorPlacement.EquallySpacedRectSide\",\"uuid\":\"60ec3ebf-862c-483f-92ed-a42ebaf3a63c\"},{\"content\":{\"connectorIds\":[\"Out1\",\"Out2\"],\"side\":\"BOTTOM\"},\"type\":\"ConnectorPlacement.EquallySpacedRectSide\",\"uuid\":\"f98c7c2b-316e-45bc-8c6b-0f1cfadaf682\"}]},\"type\":\"ConnectorPlacement.EquallySpacedConnector\",\"uuid\":\"dfbf4405-c89f-4eae-8823-64eb802242fb\"}],\"packageUris\":[\"http://schema.mathworks.com/mf0/Connector/R2020b\"],\"version\":\"1.0\"}"
  wires:
  WaterTsensor/1("    ") -> Bus Creator/2
  T<setPoint>/1 -> Control/2(Tset)
  Bus Creator/1 -> Scope/1  "T<liq>"
  PS-Simulink Converter4/1 -> Scope/2  "COP"
  PS-Simulink Converter3/1 -> Scope/3  "ePower (kW)"
  Fw [kg/s]/1 -> Control/3(Fw)
  Control/1(D) -> Bus Selector/1
  PS-Simulink Converter/1 -> Control/1(Tr)
  Bus Selector/1 -> Scope/4  "<Fw>"
  Bus Selector/2 -> Scope/5  "<Tr>"
  Bus Selector/3 -> Scope/6  "<Op>"
  Bus Selector/4 -> Scope/7  "<Vg>"
  Bus Selector/5 -> Scope/8  "<Ta>"
  WaterTsensor/2("   ") -> Bus Creator/1
  Bus Selector/6 -> Scope/9  "<Ep>"
  connections:
  Ambient/RConn2 -- Building/LConn2
  Connection Label/LConn1 -- GroundThermalResistance/RConn1
  OperationalData/LConn2 -- Thermal Liquid Settings (TL)/RConn1 -- HeatPump/RConn2 -- WaterTsensor/LConn1
  PS-Simulink Converter3/LConn1 -- HeatPump/RConn3
  PS-Simulink Converter4/LConn1 -- HeatPump/RConn4
  Control/RConn2 -- Building/LConn1 -- Ambient/RConn1 -- Connection Label1/LConn1
  Control/RConn1 -- Building/LConn3
  Control/LConn4 -- HeatPump/LConn3
  Building/RConn1 -- PS-Simulink Converter/LConn1
  Control/LConn5 -- HeatPump/LConn4
  Solver Configuration/RConn1 -- OperationalData/LConn1 -- HeatPump/RConn1 -- WaterTsensor/LConn2
  Control/LConn2 -- HeatPump/LConn1
  Control/LConn3 -- HeatPump/LConn2
  Building/RConn2 -- PS Terminator1/LConn1
  Building/RConn4 -- GroundThermalResistance/LConn1
  Control/LConn1 -- OperationalData/LConn3
  OperationalData/LConn4 -- Building/LConn4
  OperationalData/RConn1 -- Building/LConn5
  OperationalData/RConn2 -- Building/RConn3
